simulink library "range_choice"  (R2013a)
settings: Solver=ode45  StartTime=0.0  StopTime=10.0  RelTol=1e-3
undefined symbols (not defined in the file): gorch_range
libraries: range_choice x1
settings Model: Creator=Leo  LastModifiedBy=Leo

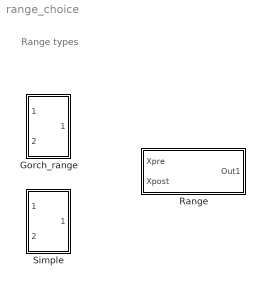
== system range_choice ==
  note: Range types
  Gorch_range : Subsystem
  Range : Subsystem  BlockChoice=Gorch_range
      settings: TemplateBlock=self  MemberBlocks=Gorch_range,Simple
  Simple : Subsystem

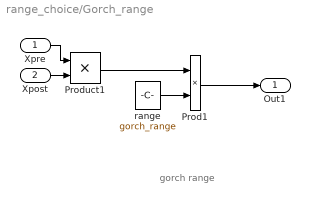
== system range_choice/Gorch_range ==
  note: gorch range
  Xpre : Inport
  Xpost : Inport  Port=2
  Prod1 : Product  RndMeth=Zero
  Product1 : Product
  range : Constant  Value=gorch_range
  Out1 : Outport
  wires:
  Product1/1 -> Prod1/1
  Xpost/1 -> Product1/2
  Prod1/1 -> Out1/1
  Xpre/1 -> Product1/1
  range/1 -> Prod1/2

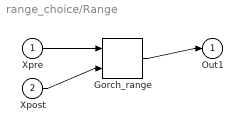
== system range_choice/Range ==
  Xpre : Inport
  Xpost : Inport  Port=2
  Gorch_range : range_choice/Gorch_range
  Out1 : Outport
  wires:
  Xpre/1 -> Gorch_range/1
  Xpost/1 -> Gorch_range/2
  Gorch_range/1 -> Out1/1

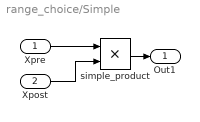
== system range_choice/Simple ==
  Xpre : Inport
  Xpost : Inport  Port=2
  simple_product : Product
  Out1 : Outport
  wires:
  simple_product/1 -> Out1/1
  Xpre/1 -> simple_product/1
  Xpost/1 -> simple_product/2
